simulink model "untitled"  (R2015b)
settings: Solver=FixedStepAuto  StartTime=0.0  StopTime=10  FixedStep=0.002  RelTol=1e-3
settings Model: ExtModeTrigDuration=5000  Creator=UFRN  LastModifiedBy=UFRN
settings SolverCC: PositivePriorityOrder=on
settings RTWCC: SystemTargetFile=quarc_win64.tlc  TemplateMakefile=quarc_default_tmf  Description=QUARC Win64 Target
settings STFCustomTargetCC: GeneratePreprocessorConditionals=Use local settings  CPPClassGenCompliant=off
settings GRTTargetCC: ParMdlRefBuildCompliant=off  CompOptLevelCompliant=off  CombineOutputUpdateFcns=off  MatFileLogging=off  CPPClassGenCompliant=off  GRTInterface=on  UseToolchainInfoCompliant=off  ExtMode=on  ExtModeMexFile=quarc_comm

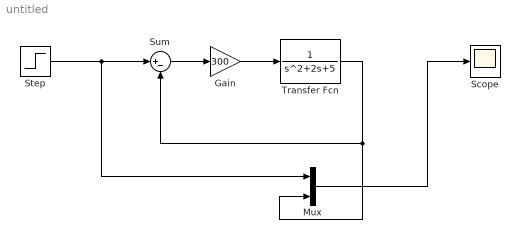
== system untitled ==
  Gain : Gain  Gain=300
  Mux : Mux  Inputs=2
  Scope : Scope
  Step : Step  Time=3  After=10  SampleTime=0
  Sum : Sum  Inputs=|+-
  Transfer Fcn : TransferFcn  Denominator=[1 2 5]
  wires:
  Transfer Fcn/1 -> Sum/2, Mux/2
  Mux/1 -> Scope/1
  Step/1 -> Mux/1, Sum/1
  Sum/1 -> Gain/1
  Gain/1 -> Transfer Fcn/1
